simulink model "sampleModel8"  (R2021b)
settings: Solver=VariableStepAuto  StartTime=0.0  StopTime=10.0  RelTol=1e-3
libraries: simulink x9
settings Model: Creator=user  LastModifiedBy=user

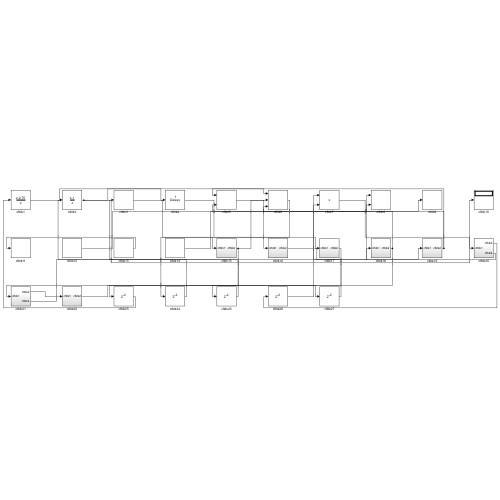
[thumbnail: Simulink's stored preview of the top-level diagram]
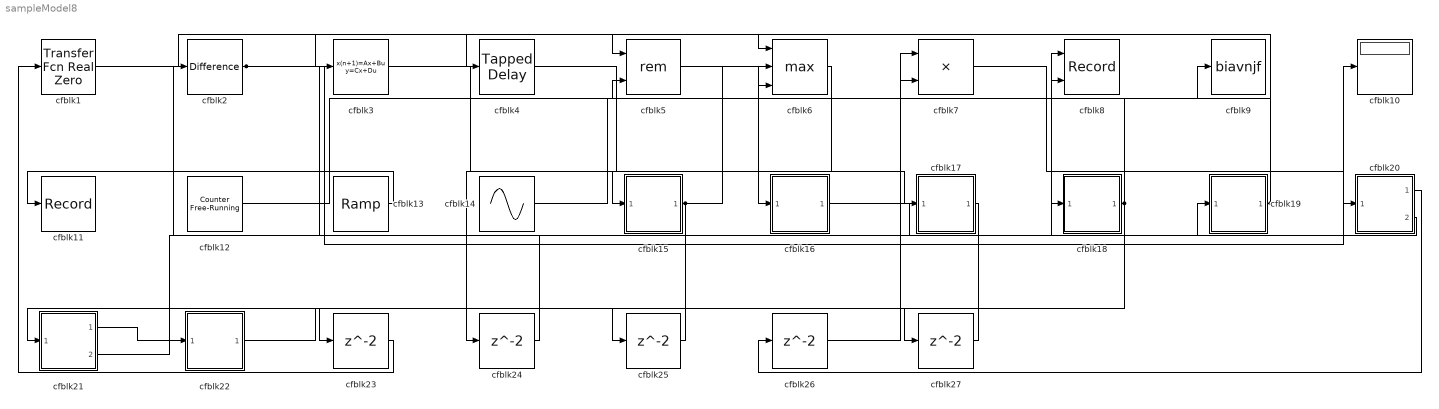
== system sampleModel8 ==
  cfblk1 : simulink/Discrete/Transfer Fcn Real Zero  ZeroZ=0.75  ICPrevInput=0.0  DoSatur=off
      settings: SourceProductBaseCode=SL
  cfblk10 : Display
  cfblk11 : Record  FileSettingsInternal="{\"entries\":[{\"content\":{\"excelSettings\":{\"content\":{},\"type\":\"Streamout.ExcelSettings\"}},\"type\":\"Streamout.FileSettingStorage\",\"uuid\":\"95cae247-3e3d-4143-a42d-d3e8033b4f95\"}],\"packageUris\":[\"http://schema.mathworks.com/mf0/streamout_blocks/R2020a\"],\"version\":\"1.0\"}"  SignalsInternal="{\"entries\":[{\"content\":{\"signals\":[{\"content\":{\"blockPath\":[\"sampleModel8/cfblk11\"],\"channel\":[],\"dimensions\":[1],\"domain\":\"sampleModel8/cfblk11\",\"lineColor\":\"#fe330a\",\"plots\":[1],\"port\":1,\"sid\":[\"\"],\"signalID\":306,\"signalName\":\"cfblk13\"},\"type\":\"RecordBlkView.Signal\",\"uuid\":\"3ee708d4-2d67-448e-8dde-6ec992259b79\"}]},\"type\":\"RecordBlkView.InputSignals\",\"uuid\":\"d1b02e5e-e756-485f-9f67-f94545486382\"}],\"packageUris\":[\"http://schema.mathworks.com/mf0/streamout_blocks/R2020a\"],\"version\":\"1.0\"}"  VisualizationBindings="{\"sparklinesplugin\":{\"info\":[{\"bindingParametersList\":[],\"subplotID\":1}]}}"
  cfblk12 : simulink/Sources/Counter Free-Running  NumBits=[32.000000]  tsamp=-1
  cfblk13 : simulink/Sources/Ramp  slope=[-4210.302672]  start=[4.350174]  InitialOutput=[-830058.508866]
  cfblk14 : Sin  Amplitude=[-863321063.731996]  Bias=[-180367001.698996]  SampleTime=0
  cfblk15 : Subsystem
  cfblk16 : Subsystem
  cfblk17 : Subsystem
  cfblk18 : Subsystem
  cfblk19 : Subsystem
  cfblk2 : simulink/Discrete/Difference  ICPrevInput=0.0  OutMin=[]  OutMax=[]  OutDataTypeStr=Inherit: Inherit via back propagation  OutDataType=fixdt(1, 16)  OutScaling=2^-10  DoSatur=off
  cfblk20 : Subsystem
  cfblk21 : Subsystem
  cfblk22 : Subsystem
  cfblk{23..27} (5 alike) : Delay  SampleTime=1
  cfblk3 : DiscreteStateSpace
  cfblk4 : simulink/Discrete/Tapped Delay  vinit=0.0  samptime=-1  NumDelays=1  DelayOrder=Oldest  includeCurrent=off
  cfblk5 : Math  Operator=rem  SaturateOnIntegerOverflow=on
  cfblk6 : MinMax  Function=max  Inputs=3
  cfblk7 : Product
  cfblk8 : Record  FileSettingsInternal="{\"entries\":[{\"content\":{\"excelSettings\":{\"content\":{},\"type\":\"Streamout.ExcelSettings\"}},\"type\":\"Streamout.FileSettingStorage\",\"uuid\":\"151b034d-9397-49e7-b2a5-d89d8af06d34\"}],\"packageUris\":[\"http://schema.mathworks.com/mf0/streamout_blocks/R2020a\"],\"version\":\"1.0\"}"  Layout=[1 1]  SignalsInternal="{\"entries\":[{\"content\":{\"signals\":[{\"content\":{\"blockPath\":[\"sampleModel8/cfblk8\"],\"channel\":[],\"dimensions\":[1],\"domain\":\"sampleModel8/cfblk8\",\"lineColor\":\"#a2142f\",\"plots\":[1],\"port\":1,\"sid\":[\"\"],\"signalID\":298,\"signalName\":\"cfblk16\"},\"type\":\"RecordBlkView.Signal\",\"uuid\":\"b0d582ed-65cd-45cc-997d-839d03a38232\"},{\"content\":{\"blockPath\":[\"sampleModel8/cfblk8\"],\"channel\":[],\"dimensions\":[1],\"domain\":\"sampleModel8/cfblk8\",\"lineColor\":\"#139fff\",\"plots\":[1],\"port\":2,\"sid\":[\"\"],\"signalID\":302,\"signalName\":\"cfblk14\"},\"type\":\"RecordBlkView.Signal\",\"uuid\":\"996b97e9-f2aa-4031-909e-f816e0eb2585\"}]},\"type\":\"RecordBlkView.InputSignals\",\"uuid\":\"b6a08acf-b630-443a-a5a4-8087fa1498da\"}],\"packageUris\":[\"http://schema.mathworks.com/mf0/streamout_blocks/R2020a\"],\"version\":\"1.0\"}"  VisualizationBindings="{\"xyplotplugin\":{\"info\":[{\"series\":[{\"bindingParametersList\":[{\"parameter\":\"X-Axis\",\"signalID\":298,\"signalName\":\"cfblk16\"},{\"parameter\":\"Y-Axis\",\"signalID\":302,\"signalName\":\"cfblk14\"}],\"seriesID\":54853}],\"subplotID\":1}]}}"  CompatibilityTag=XY
  cfblk9 : ToWorkspace  VariableName=biavnjf  SaveFormat=Timeseries  SampleTime=-1
  wires:
  cfblk3/1 -> cfblk15/1(cfblk1)
  cfblk5/1 -> cfblk16/1(cfblk1)
  cfblk16/1(cfblk2) -> cfblk8/1
  cfblk2/1 -> cfblk10/1, cfblk6/1
  cfblk1/1 -> cfblk4/1
  cfblk14/1 -> cfblk8/2
  cfblk19/1(cfblk2) -> cfblk5/1, cfblk5/2
  cfblk21/1(cfblk2) -> cfblk22/1(cfblk1)
  cfblk15/1(cfblk2) -> cfblk6/2, cfblk25/1
  cfblk7/1 -> cfblk20/1(cfblk1)
  cfblk21/2(cfblk4) -> cfblk19/1(cfblk1)
  cfblk4/1 -> cfblk17/1(cfblk1)
  cfblk13/1 -> cfblk11/1
  cfblk12/1 -> cfblk9/1
  cfblk18/1(cfblk2) -> cfblk21/1(cfblk1), cfblk6/3
  cfblk20/2(cfblk4) -> cfblk18/1(cfblk1)
  cfblk17/1(cfblk2) -> cfblk23/1
  cfblk23/1 -> cfblk1/1
  cfblk6/1 -> cfblk24/1
  cfblk24/1 -> cfblk2/1
  cfblk25/1 -> cfblk3/1
  cfblk20/1(cfblk2) -> cfblk26/1
  cfblk26/1 -> cfblk7/2
  cfblk22/1(cfblk2) -> cfblk27/1
  cfblk27/1 -> cfblk7/1

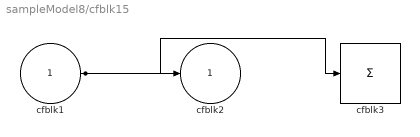
== system sampleModel8/cfblk15 ==
  cfblk1 : Inport
  cfblk3 : Sum  Inputs=+
  cfblk2 : Outport
  wires:
  cfblk1/1 -> cfblk2/1, cfblk3/1

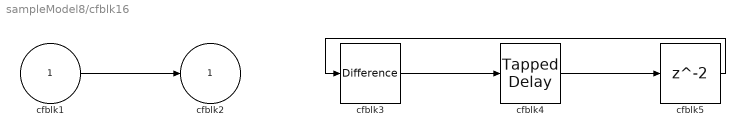
== system sampleModel8/cfblk16 ==
  cfblk1 : Inport
  cfblk3 : simulink/Discrete/Difference  ICPrevInput=0.0  OutMin=[]  OutMax=[]  OutDataTypeStr=Inherit: Inherit via back propagation  OutDataType=fixdt(1, 16)  OutScaling=2^-10  DoSatur=off
  cfblk4 : simulink/Discrete/Tapped Delay  vinit=0.0  samptime=-1  NumDelays=1  DelayOrder=Oldest  includeCurrent=off
  cfblk5 : Delay  SampleTime=1
  cfblk2 : Outport
  wires:
  cfblk3/1 -> cfblk4/1
  cfblk1/1 -> cfblk2/1
  cfblk4/1 -> cfblk5/1
  cfblk5/1 -> cfblk3/1

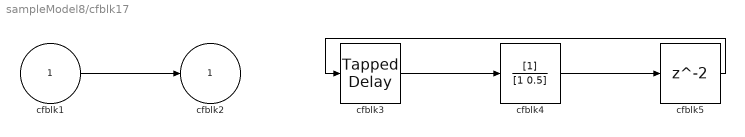
== system sampleModel8/cfblk17 ==
  cfblk1 : Inport
  cfblk3 : simulink/Discrete/Tapped Delay  vinit=0.0  samptime=-1  NumDelays=1  DelayOrder=Oldest  includeCurrent=off
  cfblk4 : DiscreteFilter  SampleTime=1
  cfblk5 : Delay  SampleTime=1
  cfblk2 : Outport
  wires:
  cfblk3/1 -> cfblk4/1
  cfblk1/1 -> cfblk2/1
  cfblk4/1 -> cfblk5/1
  cfblk5/1 -> cfblk3/1

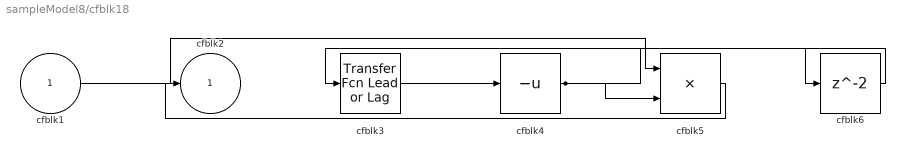
== system sampleModel8/cfblk18 ==
  cfblk1 : Inport
  cfblk3 : simulink/Discrete/Transfer Fcn Lead or Lag  PoleZ=0.95  ZeroZ=0.75  ICPrevOutput=0.0  ICPrevInput=0.0  DoSatur=off
      settings: SourceProductBaseCode=SL
  cfblk4 : UnaryMinus
  cfblk5 : Product  Inputs=**
  cfblk6 : Delay  SampleTime=1
  cfblk2 : Outport
  wires:
  cfblk4/1 -> cfblk5/2, cfblk6/1
  cfblk3/1 -> cfblk4/1
  cfblk1/1 -> cfblk5/1
  cfblk5/1 -> cfblk2/1
  cfblk6/1 -> cfblk3/1

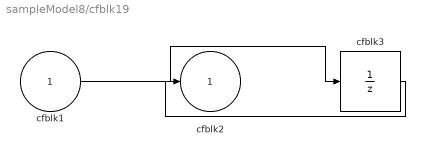
== system sampleModel8/cfblk19 ==
  cfblk1 : Inport
  cfblk3 : UnitDelay  HasFrameUpgradeWarning=on
  cfblk2 : Outport
  wires:
  cfblk1/1 -> cfblk3/1
  cfblk3/1 -> cfblk2/1

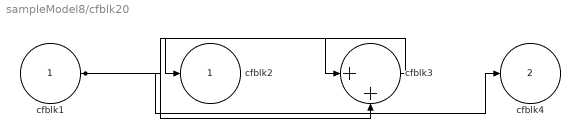
== system sampleModel8/cfblk20 ==
  cfblk1 : Inport
  cfblk3 : Sum  Inputs=|++
  cfblk2 : Outport
  cfblk4 : Outport  Port=2
  wires:
  cfblk3/1 -> cfblk2/1
  cfblk1/1 -> cfblk4/1, cfblk3/1, cfblk3/2

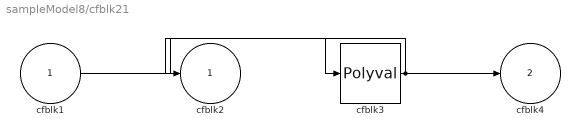
== system sampleModel8/cfblk21 ==
  cfblk1 : Inport
  cfblk3 : Polyval  Coefs=[ +2.081618890e-019, -1.441693666e-014, +4.719686976e-010, -8.536869453e-006, +1.621573104e-001, -8.087801117e+001 ]
  cfblk2 : Outport
  cfblk4 : Outport  Port=2
  wires:
  cfblk1/1 -> cfblk3/1
  cfblk3/1 -> cfblk4/1, cfblk2/1

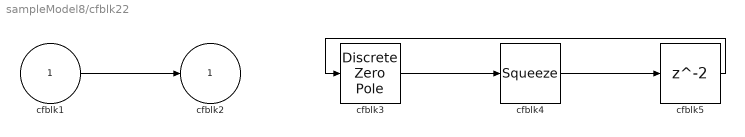
== system sampleModel8/cfblk22 ==
  cfblk1 : Inport
  cfblk3 : DiscreteZeroPole  Poles=[0 0.5]  Gain=1
  cfblk4 : Squeeze
  cfblk5 : Delay  SampleTime=1
  cfblk2 : Outport
  wires:
  cfblk3/1 -> cfblk4/1
  cfblk1/1 -> cfblk2/1
  cfblk4/1 -> cfblk5/1
  cfblk5/1 -> cfblk3/1
